simulink model "ODE1_zad3"  (Simulink 6.3)
settings: Solver=ode45  StartTime=0.0  StopTime=0.4  RelTol=1e-3
settings Model: LastModifiedBy=Ms1

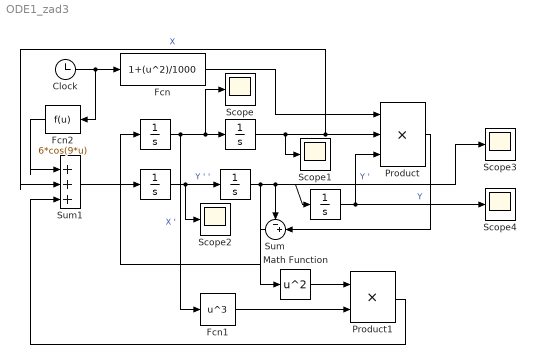
== system ODE1_zad3 ==
  " " : Integrator  InitialCondition=95
  "   " : Integrator  InitialCondition=11
  "    " : Integrator  InitialCondition=-2
  "       " : Integrator
  "           " : Integrator  InitialCondition=7
  Clock : Clock
      settings: Decimation=10
  Fcn : Fcn  Expr=1+(u^2)/1000
  Fcn1 : Fcn  Expr=u^3
  Fcn2 : Fcn  Orientation=left  Expr=6*cos(9*u)
  Math Function : Math  Operator=square  SaturateOnIntegerOverflow=on
  Product : Product  Inputs=3  SaturateOnIntegerOverflow=on  InputSameDT=on
  Product1 : Product  SaturateOnIntegerOverflow=on  InputSameDT=on
  Scope{,1..4} (5 alike) : Scope
      Scope2 settings: SaveName=ScopeData2
      Scope3 settings: SaveName=ScopeData3
      Scope4 settings: SaveName=ScopeData4
  Sum : Sum  Orientation=left  Inputs=-+|  SaturateOnIntegerOverflow=on  InputSameDT=on
  Sum1 : Sum  Inputs=|+++  SaturateOnIntegerOverflow=on  InputSameDT=on
  wires:
  " "/1 -> "   "/1, Scope2/1  "Y ' '"
  "   "/1 -> Scope3/1, Sum/1, "    "/1, Math Function/1  "Y '"
  "       "/1 -> Fcn1/1, "           "/1, Scope/1  "X '"
  Clock/1 -> Fcn/1, Fcn2/1
  Fcn/1 -> Product/1
  "           "/1 -> Product/2, Sum1/2, Scope1/1  "X"
  "    "/1 -> Product/3, Scope4/1  "Y"
  Product/1 -> Sum/2
  Sum/1 -> "       "/1
  Math Function/1 -> Product1/1
  Fcn1/1 -> Product1/2
  Fcn2/1 -> Sum1/1
  Sum1/1 -> " "/1
  Product1/1 -> Sum1/3
